simulink model "hCVT"  (R2025a)
settings: Solver=VariableStepAuto  StartTime=0.0  StopTime=10  RelTol=1e-3
InitFcn:
  | WLTP
  | BSFC
  | Vehicle
values from neighbouring files (symbols this model uses):
  A = 2.2    [Main.m]    (also in Main_cvt.m; PlotCVT_new.m = data{:,1}; Vehicle.m; cvtka.m)
  Cd = 0.32    [Main.m]    (also in Main_cvt.m; Vehicle.m; cvtka.m = 0.31)
  Cr = 0.015    [Main.m]    (also in Main_cvt.m; Vehicle.m; cvtka.m = 0.012)
  g = 9.81    [Main.m]    (also in Main_cvt.m; Vehicle.m; cvtka.m)
  m = 1600    [Main.m]    (also in Main_cvt.m; Vehicle.m; cvtka.m = 1250)
  r = 0.285    [Main.m]    (also in Main_cvt.m; Vehicle.m; cvtka.m)
  rho = 1.225    [Main.m]    (also in Main_cvt.m; Vehicle.m; cvtka.m)
settings Model: Creator=Admin  LastModifiedBy=Admin

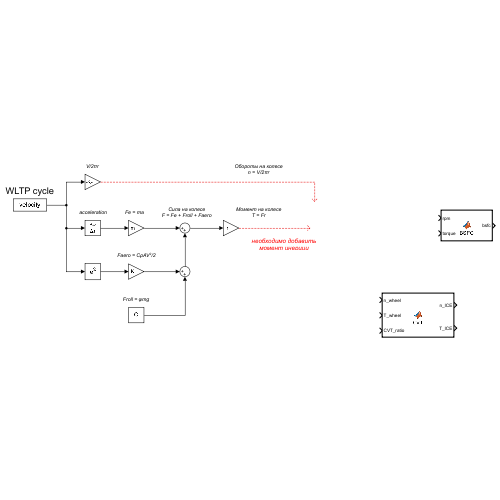
[thumbnail: Simulink's stored preview of the top-level diagram]
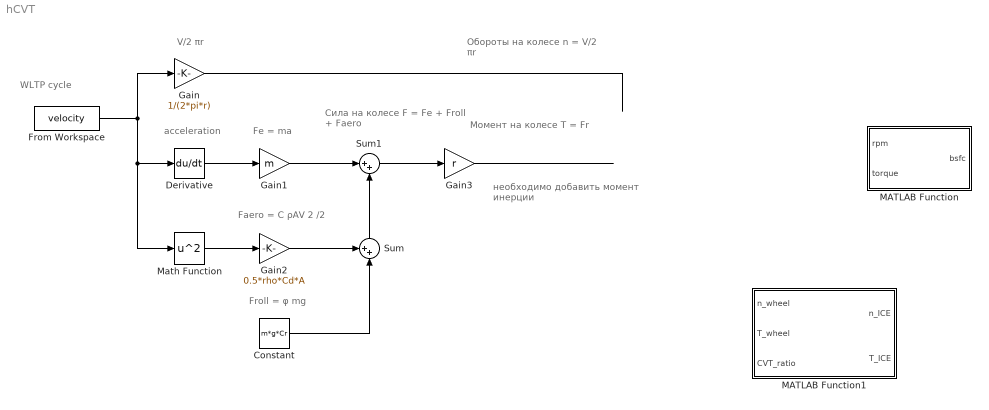
== system hCVT ==
  note: acceleration
  note: WLTP cycle
  note: V/2 πr
  note: Fe = ma
  note: Froll = φ mg
  note: Faero = C ρAV 2 /2
  note: Сила на колесе
      | F = Fe + Froll + Faero
  note: Момент на колесе
      | T = Fr
  note: Обороты на колесе
      | n = V/2 πr
  note: необходимо добавить момент инерции
  Constant : Constant  Value=m*g*Cr
  Derivative : Derivative
  From Workspace : FromWorkspace  VariableName=velocity
  Gain : Gain  Gain=1/(2*pi*r)
  Gain1 : Gain  Gain=m
  Gain2 : Gain  Gain=0.5*rho*Cd*A
  Gain3 : Gain  Gain=r
  MATLAB Function : MATLAB Function  TreatAsAtomicUnit=on
  MATLAB Function1 : MATLAB Function  TreatAsAtomicUnit=on
  Math Function : Math  Operator=square
  Sum : Sum  Inputs=++|
  Sum1 : Sum  Inputs=|++
  wires:
  From Workspace/1 -> Gain/1, Derivative/1, Math Function/1
  Derivative/1 -> Gain1/1
  Math Function/1 -> Gain2/1
  Gain2/1 -> Sum/1
  Constant/1 -> Sum/2
  Gain1/1 -> Sum1/1
  Sum/1 -> Sum1/2
  Sum1/1 -> Gain3/1
  Gain/1 -> ?
  Gain3/1 -> ?

== matlab function hCVT/MATLAB Function1 ==
  data: n_ICE output; n_wheel input; T_ICE output; T_wheel input; CVT_ratio input
function [n_ICE, T_ICE] = CVT(n_wheel, T_wheel, CVT_ratio)

% параметры из workspace
vehicle = evalin('base','vehicle');

            % ------ %    главная передача     % ------ %

% обороты до ГП
n_GP = n_wheel * GP_ratio;

% момент до ГП
T_GP = T_wheel/(GP_ratio * GP_efficiency);

                % ------ %    вариатор     % ------ %

CVT_efficiency = eta_CVT(n_GP, T_GP);

% обороты до ГП
n_ICE = n_GP * CVT_ratio;

% момент до ГП
T_ICE = T_GP/(CVT_ratio * CVT_efficiency);
     
end

== matlab function hCVT/MATLAB Function ==
  data: rpm input; bsfc output; torque input
function bsfc = BSFC(rpm, torque)
    % BSFC интерполяция по триангулированной поверхности
    % Получаем обороты и момент -> находим треугольник -> интерполируем
    
    persistent vertices triangles
    persistent rpm_min rpm_max torque_min torque_max
    persistent nTri
    
    % Загружаем данные при первом вызове
    if isempty(vertices)
        S = coder.load('BSFC_surface.mat');
        vertices = S.all_vertices;
        triangles = S.all_triangles;
        
        rpm_min = min(vertices(:,1));
        rpm_max = max(vertices(:,1));
        torque_min = min(vertices(:,2));
        torque_max = max(vertices(:,2));
        
        nTri = size(triangles, 1);
    end
    
    % Проверяем, что точка внутри области данных
    if rpm < rpm_min || rpm > rpm_max || torque < torque_min || torque > torque_max
        % Точка вне области - возвращаем NaN или можно задать граничное значение
        bsfc = NaN;
        return;
    end
    
    % Ищем треугольник, содержащий точку
    for t = 1:nTri
        % Получаем вершины треугольника
        i1 = triangles(t, 1);
        i2 = triangles(t, 2);
        i3 = triangles(t, 3);
        
        p1 = vertices(i1, :);
        p2 = vertices(i2, :);
        p3 = vertices(i3, :);
        
        % Проверяем, находится ли точка внутри треугольника
        if pointInTriangle([rpm, torque], p1(1:2), p2(1:2), p3(1:2))
            % Точка внутри - делаем барицентрическую интерполяцию
            bsfc = barycentricInterp(p1, p2, p3, [rpm, torque]);
            return;
        end
    end
    
    % Если не нашли треугольник (точка между контурами, но вне треугольников)
    % Такое возможно на границах между уровнями
    bsfc = NaN;
end

function inside = pointInTriangle(pt, p1, p2, p3)
    % Проверка, находится ли точка внутри треугольника
    % pt, p1, p2, p3 - точки [x y]
    
    % Вычисляем барицентрические координаты
    v0 = p3 - p1;
    v1 = p2 - p1;
    v2 = pt - p1;
    
    dot00 = v0(1)*v0(1) + v0(2)*v0(2);
    dot01 = v0(1)*v1(1) + v0(2)*v1(2);
    dot02 = v0(1)*v2(1) + v0(2)*v2(2);
    dot11 = v1(1)*v1(1) + v1(2)*v1(2);
    dot12 = v1(1)*v2(1) + v1(2)*v2(2);
    
    invDenom = 1 / (dot00 * dot11 - dot01 * dot01);
    u = (dot11 * dot02 - dot01 * dot12) * invDenom;
    v = (dot00 * dot12 - dot01 * dot02) * invDenom;
    
    % Проверка: точка внутри, если u >= 0, v >= 0 и u + v <= 1
    inside = (u >= 0) && (v >= 0) && (u + v <= 1);
end

function z = barycentricInterp(p1, p2, p3, pt)
    % Барицентрическая интерполяция для получения Z
    % p1, p2, p3 - вершины треугольника [x y z]
    % pt - точка [x y]
    
    % Вычисляем барицентрические координаты
    v0 = p3(1:2) - p1(1:2);
    v1 = p2(1:2) - p1(1:2);
    v2 = pt - p1(1:2);
    
    dot00 = v0(1)*v0(1) + v0(2)*v0(2);
    dot01 = v0(1)*v1(1) + v0(2)*v1(2);
    dot02 = v0(1)*v2(1) + v0(2)*v2(2);
    dot11 = v1(1)*v1(1) + v1(2)*v1(2);
    dot12 = v1(1)*v2(1) + v1(2)*v2(2);
    
    invDenom = 1 / (dot00 * dot11 - dot01 * dot01);
    u = (dot11 * dot02 - dot01 * dot12) * invDenom;
    v = (dot00 * dot12 - dot01 * dot02) * invDenom;
    w = 1 - u - v;
    
    % Интерполяция Z
    z = w * p1(3) + v * p2(3) + u * p3(3);
end
